simulink model "TST_RailP_VDSync"  (R2016b)
settings: Solver=FixedStepDiscrete  StartTime=0.0  StopTime=simTime  FixedStep=sampleTime  RelTol=1e-3
values from neighbouring files (symbols this model uses):
  testCase = 1    [initTST_RailP_VDSync_001.m]
libraries: simulink x3, UnitTest_Lib x1
settings Model: Creator=zhengjinyan  LastModifiedBy=zhengjinyan
settings DebuggingCC: SignalRangeChecking=error

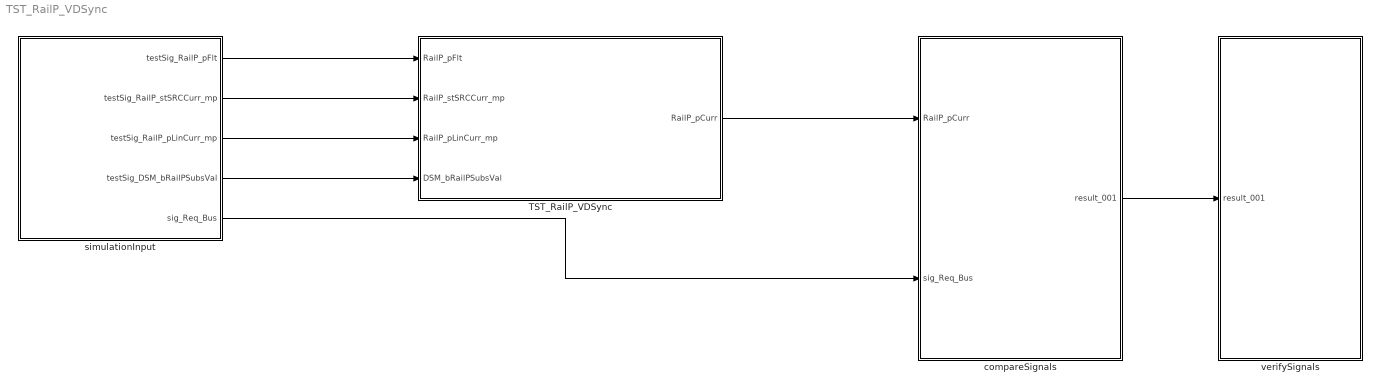
== system TST_RailP_VDSync ==
  TST_RailP_VDSync : Subsystem
  compareSignals : Subsystem
  simulationInput : Subsystem
  verifySignals : Subsystem
  wires:
  simulationInput/1(testSig_RailP_pFlt) -> TST_RailP_VDSync/1(RailP_pFlt)
  simulationInput/2(testSig_RailP_stSRCCurr_mp) -> TST_RailP_VDSync/2(RailP_stSRCCurr_mp)
  simulationInput/3(testSig_RailP_pLinCurr_mp) -> TST_RailP_VDSync/3(RailP_pLinCurr_mp)
  simulationInput/4(testSig_DSM_bRailPSubsVal) -> TST_RailP_VDSync/4(DSM_bRailPSubsVal)
  TST_RailP_VDSync/1(RailP_pCurr) -> compareSignals/1(RailP_pCurr)
  simulationInput/5(sig_Req_Bus) -> compareSignals/2(sig_Req_Bus)
  compareSignals/1(result_001) -> verifySignals/1(result_001)

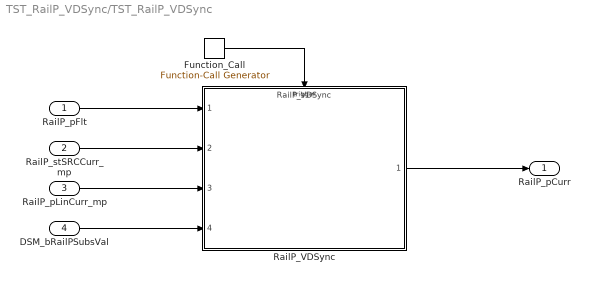
== system TST_RailP_VDSync/TST_RailP_VDSync ==
  RailP_pFlt : Inport
  RailP_stSRCCurr_mp : Inport  Port=2
  RailP_pLinCurr_mp : Inport  Port=3
  DSM_bRailPSubsVal : Inport  Port=4
  Function_Call : simulink/Ports & Subsystems/Function-Call Generator  sample_time=sampleTime  numberOfIterations=1
  RailP_VDSync : ModelReference  ModelNameDialog=RailP_VDSync  SimulationMode=Normal  ModelReferenceVersion=1.3  TriggerPortName=function  TriggerPortTriggerType=function-call  TriggerPortStatesWhenEnabling=held
  RailP_pCurr : Outport
  wires:
  Function_Call/1 -> RailP_VDSync/Trigger
  RailP_pFlt/1 -> RailP_VDSync/1
  RailP_stSRCCurr_mp/1 -> RailP_VDSync/2
  RailP_pLinCurr_mp/1 -> RailP_VDSync/3
  DSM_bRailPSubsVal/1 -> RailP_VDSync/4
  RailP_VDSync/1 -> RailP_pCurr/1

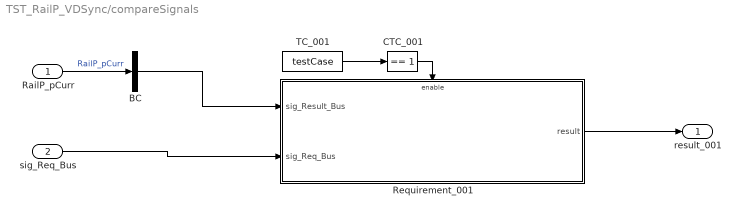
== system TST_RailP_VDSync/compareSignals ==
  RailP_pCurr : Inport
  sig_Req_Bus : Inport  Port=2
  BC : BusCreator  Inputs=1
  CTC_001 : simulink/Logic and Bit Operations/Compare To Constant  relop===  const=1  OutDataTypeStr=boolean
  Requirement_001 : Subsystem
  TC_001 : Constant  Value=testCase
  result_001 : Outport
  wires:
  RailP_pCurr/1 -> BC/1  "RailP_pCurr"
  TC_001/1 -> CTC_001/1
  CTC_001/1 -> Requirement_001/Enable
  sig_Req_Bus/1 -> Requirement_001/2(sig_Req_Bus)
  BC/1 -> Requirement_001/1(sig_Result_Bus)
  Requirement_001/1(result) -> result_001/1

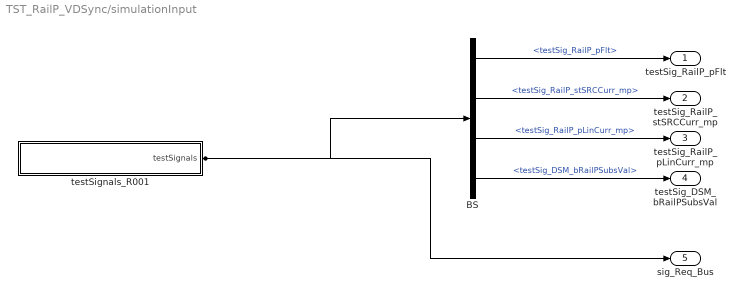
== system TST_RailP_VDSync/simulationInput ==
  BS : BusSelector  OutputSignals=testSig_RailP_pFlt,testSig_RailP_stSRCCurr_mp,testSig_RailP_pLinCurr_mp,testSig_DSM_bRailPSubsVal
  testSignals_R001 : Subsystem
  testSig_RailP_pFlt : Outport
  testSig_RailP_stSRCCurr_mp : Outport  Port=2
  testSig_RailP_pLinCurr_mp : Outport  Port=3
  testSig_DSM_bRailPSubsVal : Outport  Port=4
  sig_Req_Bus : Outport  Port=5
  wires:
  BS/1 -> testSig_RailP_pFlt/1  "<testSig_RailP_pFlt>"
  BS/2 -> testSig_RailP_stSRCCurr_mp/1  "<testSig_RailP_stSRCCurr_mp>"
  BS/3 -> testSig_RailP_pLinCurr_mp/1  "<testSig_RailP_pLinCurr_mp>"
  BS/4 -> testSig_DSM_bRailPSubsVal/1  "<testSig_DSM_bRailPSubsVal>"
  testSignals_R001/1(testSignals) -> BS/1, sig_Req_Bus/1

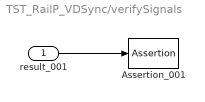
== system TST_RailP_VDSync/verifySignals ==
  result_001 : Inport
  Assertion_001 : Assertion  Enabled=off
  wires:
  result_001/1 -> Assertion_001/1

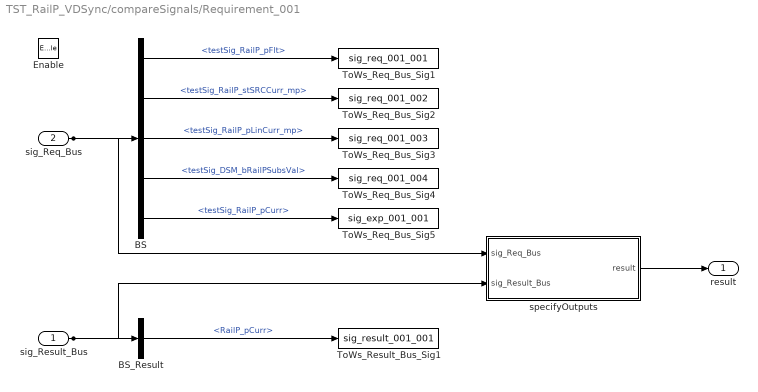
== system TST_RailP_VDSync/compareSignals/Requirement_001 ==
  sig_Result_Bus : Inport
  sig_Req_Bus : Inport  Port=2
  Enable : EnablePort
  BS : BusSelector  OutputSignals=testSig_RailP_pFlt,testSig_RailP_stSRCCurr_mp,testSig_RailP_pLinCurr_mp,testSig_DSM_bRailPSubsVal,testSig_RailP_pCurr
  BS_Result : BusSelector  OutputSignals=RailP_pCurr
  ToWs_Req_Bus_Sig1 : ToWorkspace  VariableName=sig_req_001_001  SaveFormat=Structure With Time
  ToWs_Req_Bus_Sig2 : ToWorkspace  VariableName=sig_req_001_002  SaveFormat=Structure With Time
  ToWs_Req_Bus_Sig3 : ToWorkspace  VariableName=sig_req_001_003  SaveFormat=Structure With Time
  ToWs_Req_Bus_Sig4 : ToWorkspace  VariableName=sig_req_001_004  SaveFormat=Structure With Time
  ToWs_Req_Bus_Sig5 : ToWorkspace  VariableName=sig_exp_001_001  SaveFormat=Structure With Time
  ToWs_Result_Bus_Sig1 : ToWorkspace  VariableName=sig_result_001_001  SaveFormat=Structure With Time
  specifyOutputs : Subsystem
  result : Outport
  wires:
  sig_Req_Bus/1 -> BS/1, specifyOutputs/1(sig_Req_Bus)
  BS/1 -> ToWs_Req_Bus_Sig1/1  "<testSig_RailP_pFlt>"
  BS/2 -> ToWs_Req_Bus_Sig2/1  "<testSig_RailP_stSRCCurr_mp>"
  BS/3 -> ToWs_Req_Bus_Sig3/1  "<testSig_RailP_pLinCurr_mp>"
  BS/4 -> ToWs_Req_Bus_Sig4/1  "<testSig_DSM_bRailPSubsVal>"
  BS/5 -> ToWs_Req_Bus_Sig5/1  "<testSig_RailP_pCurr>"
  sig_Result_Bus/1 -> BS_Result/1, specifyOutputs/2(sig_Result_Bus)
  BS_Result/1 -> ToWs_Result_Bus_Sig1/1  "<RailP_pCurr>"
  specifyOutputs/1(result) -> result/1

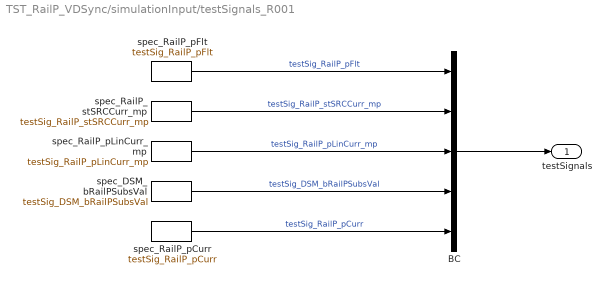
== system TST_RailP_VDSync/simulationInput/testSignals_R001 ==
  BC : BusCreator  Inputs=5
  spec_DSM_bRailPSubsVal : FromWorkspace  VariableName=testSig_DSM_bRailPSubsVal  Interpolate=off  OutputAfterFinalValue=Holding final value
  spec_RailP_pCurr : FromWorkspace  VariableName=testSig_RailP_pCurr  Interpolate=off  OutputAfterFinalValue=Holding final value
  spec_RailP_pFlt : FromWorkspace  VariableName=testSig_RailP_pFlt  Interpolate=off  OutputAfterFinalValue=Holding final value
  spec_RailP_pLinCurr_mp : FromWorkspace  VariableName=testSig_RailP_pLinCurr_mp  Interpolate=off  OutputAfterFinalValue=Holding final value
  spec_RailP_stSRCCurr_mp : FromWorkspace  VariableName=testSig_RailP_stSRCCurr_mp  Interpolate=off  OutputAfterFinalValue=Holding final value
  testSignals : Outport
  wires:
  BC/1 -> testSignals/1
  spec_RailP_pFlt/1 -> BC/1  "testSig_RailP_pFlt"
  spec_RailP_stSRCCurr_mp/1 -> BC/2  "testSig_RailP_stSRCCurr_mp"
  spec_RailP_pLinCurr_mp/1 -> BC/3  "testSig_RailP_pLinCurr_mp"
  spec_DSM_bRailPSubsVal/1 -> BC/4  "testSig_DSM_bRailPSubsVal"
  spec_RailP_pCurr/1 -> BC/5  "testSig_RailP_pCurr"

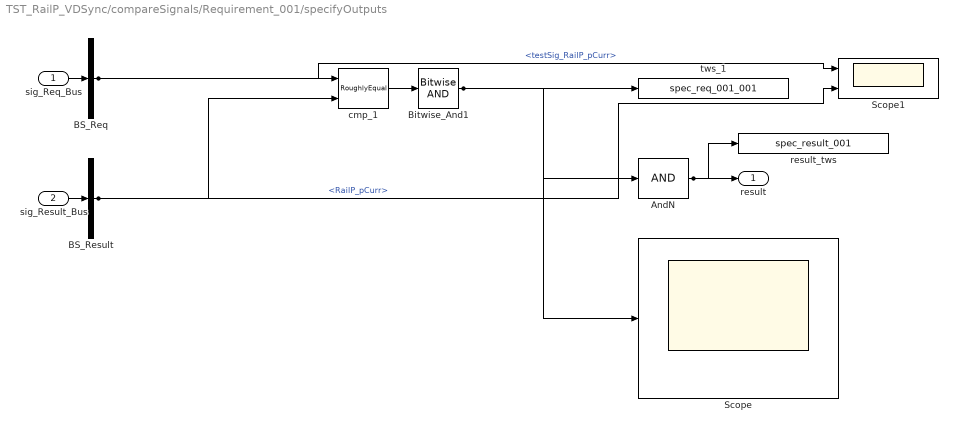
== system TST_RailP_VDSync/compareSignals/Requirement_001/specifyOutputs ==
  sig_Req_Bus : Inport
  sig_Result_Bus : Inport  Port=2
  AndN : Logic  Inputs=1
  BS_Req : BusSelector  OutputSignals=testSig_RailP_pCurr
  BS_Result : BusSelector  OutputSignals=RailP_pCurr
  Bitwise_And1 : simulink/Logic and Bit Operations/Bitwise Operator  logicop=AND  UseBitMask=off  BitMask=bin2dec('11011001')  BitMaskRealWorld=Stored Integer
  Scope : Scope
  Scope1 : Scope  NumInputPorts=2
  cmp_1 : UnitTest_Lib/RoughlyEqual  slope=0.1
  result_tws : ToWorkspace  VariableName=spec_result_001
  tws_1 : ToWorkspace  VariableName=spec_req_001_001
  result : Outport
  wires:
  sig_Req_Bus/1 -> BS_Req/1
  sig_Result_Bus/1 -> BS_Result/1
  AndN/1 -> result/1, result_tws/1
  BS_Req/1 -> cmp_1/1, Scope1/1  "<testSig_RailP_pCurr>"
  BS_Result/1 -> cmp_1/2, Scope1/2  "<RailP_pCurr>"
  cmp_1/1 -> Bitwise_And1/1
  Bitwise_And1/1 -> tws_1/1, AndN/1, Scope/1
